simulink model "aeroblk_HL20_UE"  (R2023a)
settings: Solver=ode45  StartTime=0.0  StopTime=70  RelTol=1e-3  EnableMultiTasking=on
PreLoadFcn:
  | aeroblk_init_HL20
values from neighbouring files (symbols this model uses):
  Act2Aero = 0.5*[1 -1 0 0 0 0 0;1 1 0 0 0 0 0 ;0 0 0 0 0 0 2;0 0 1 1 0 0 0; 0 0 0 0 1 1 0;0 0 1 -1 1 -1 0;]    [aeroblk_init_HL20.m]
  Aero2Act = pinv(Act2Aero)    [aeroblk_init_HL20.m]
  Aimpoint = 0    [aeroblk_init_HL20.m]
undefined symbols (not defined in the file or in its folder): alpha0, ft, hglide, m, qbar0, s, U_trim_matrix, Xglide
libraries: aerolibconvert2 x11, aeroblk_lib_HL20 x5, simulink x2, aerolibactuator x1, aerolibsim3d x1, sim3dlib x1
Description:
  | HL-20 with Simulink 3D Animation and Flight Instrumentation Blocks
  | 
  | This model shows NASA's HL-20 lifting body and controller modeled in Simulink(R),
  |  Aerospace Blockset(TM), and Simulink(R) 3D Animation(TM) software. This model simulates
  | approach and landing flight phases using an auto-landing controller. The Visualization subsystem uses
  | aircraft-specific gauges from the Aerospace Blockset(TM) Flight Instrumentation library.
  | 
  | The HL-20 also known as personnel launch system (PLS) is a lifting body re-entry
  | vehicle that was designed to complement the Space Shuttle orbiter. Designed to
  | carry up to ten people and very little cargo[1], the HL-20 lifting body was to be
  | placed in orbit either launched vertically via booster rockets or transported in the
  | payload bay of the Space Shuttle orbiter. HL-20 lifting body was designed to have a
  | powered deorbiting accomplished with an onboard propulsion system while its reentry
  | was to be nose-first, horizontal and unpowered.
  | 
  | The HL-20 lifting body was developed as a low cost solution for getting to and from
  | low Earth orbit. The proposed benefits of the HL-20 were reduced operating costs
  | due to rapid turnaround between landing and launch, improved flight safety, and
  | ability to land conventionally on runways. Potential scenarios for the HL-20 were
  | orbital rescue of stranded astronauts, International Space Station crew exchange
  | if the Space Shuttle orbiter was not available, observation missions, and satellite
  | servicing missions.
  | 
  | Additional information about HL-20
  | 
  | [1] Jackson E. B., Cruz C. L., "Preliminary Subsonic Aerodynamic Model for Simulation Studies of the HL-20 Lifting Body," NASA TM4302 (August 1992)
settings Model: ModifiedByFormat=rhyde  ModifiedComment=rhyde -- Wed Mar 13 13:42:21 2002 -- Version 1.0  ModifiedHistory=A.N.Other -- Wed Mar 13 13:42:21 2002 -- Version 1.0  Creator=The MathWorks, Inc.  LastModifiedBy=rhyde
settings SolverCC: AlgebraicLoopSolver=TrustRegion  MaxZcPerStep=1
settings DataIOCC: LimitDataPoints=on  SaveFormat=Array  ReturnWorkspaceOutputs=off  SignalLoggingName=sigsOut
settings OptimizationCC: DefaultParameterBehavior=Inlined  InlineInvariantSignals=on  ReuseModelBlockBuffer=off  ExpressionDepthLimit=2147483647  InitFltsAndDblsToZero=on  EfficientFloat2IntCast=on  LifeSpan=inf
settings DebuggingCC: SaveWithParameterizedLinksMsg=none  CheckExecutionContextPreStartOutputMsg=on  MultiTaskCondExecSysMsg=none  SigSpecEnsureSampleTimeMsg=none  FcnCallInpInsideContextMsg=warning  UnconnectedInputMsg=warning  UnconnectedOutputMsg=warning  UnconnectedLineMsg=warning  UniqueDataStoreMsg=error  AllowSymbolicDim=off  StateNameClashWarn=warning  StrictBusMsg=ErrorOnBusTreatedAsVector  SFUnexpectedBacktrackingDiag=warning  SFNoUnconditionalDefaultTransitionDiag=warning  SFExecutionAtInitializationDiag=none  ArithmeticOperatorsInVariantConditions=warning
settings HardwareCC: ProdBitPerPointer=32  ProdBitPerSizeT=32  ProdBitPerPtrDiffT=32  ProdLargestAtomicFloat=None  ProdIntDivRoundTo=Undefined  ProdEndianess=Unspecified  ProdWordSize=32  ProdHWDeviceType=32-bit Generic  TargetUnknown=on
settings ModelReferenceCC: EnableRefExpFcnMdlSchedulingChecks=on  PropagateSignalLabelsOutOfModel=off
settings SFSimCC: SimUseLocalCustomCode=off  CustomCodeUndefinedFunction=UseInterfaceOnly
settings RTWCC: RTWUseLocalCustomCode=off  DLArmComputeVersion=19.05
settings CodeAppCC: StateflowObjectComments=on
settings GRTTargetCC: TargetFcnLib=ansi_tfl_tmw.mat  TargetLangStandard=C89/C90 (ANSI)  CombineOutputUpdateFcns=off  GRTInterface=on
settings ConfigComp: CovMetricSettings=dw  CovSaveCumulativeToWorkspaceVar=on  CovSaveSingleToWorkspaceVar=on  CovExternalEMLEnable=off

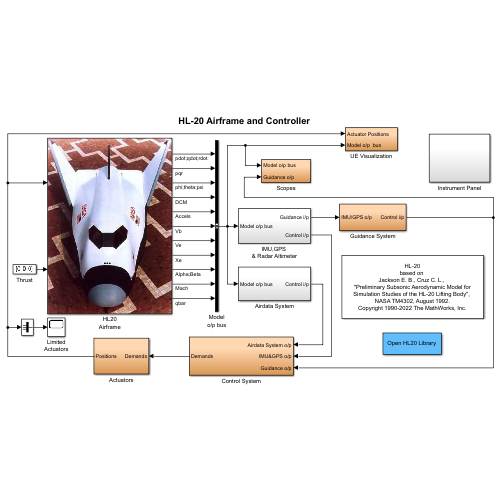
[thumbnail: Simulink's stored preview of the top-level diagram]
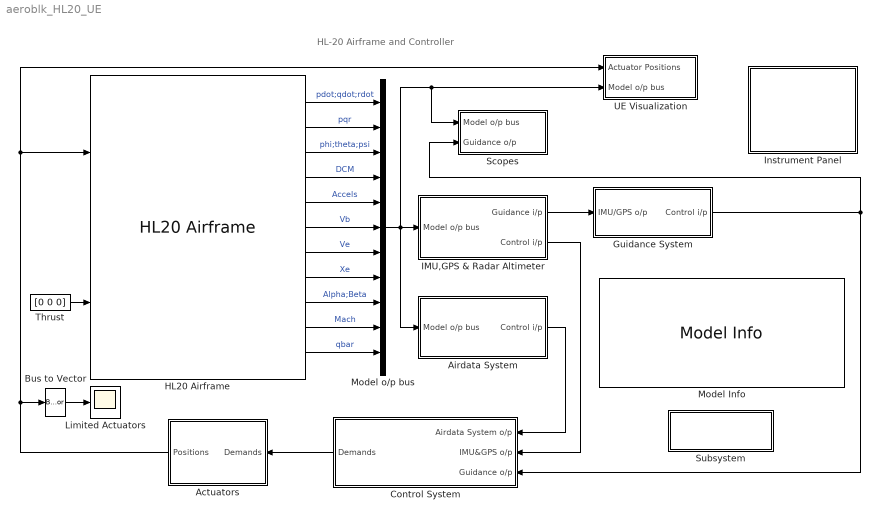
== system aeroblk_HL20_UE ==
  note: HL-20 Airframe and Controller
  Actuators : Subsystem
  Airdata System : Subsystem
  Bus to Vector : BusToVector
  Control System : Subsystem
  Guidance System : Subsystem
  HL20 Airframe : aeroblk_lib_HL20/HL20 Airframe  SystemSampleTime=-1  VariantActivationTime=update diagram  Latency=0  AutoFrameSizeCalculation=off
  IMU,GPS & Radar Altimeter : Subsystem
  Instrument Panel : Subsystem
  Limited Actuators : Scope
  Model o/p bus : BusCreator  Inputs=11
  Model Info : simulink/Model-Wide Utilities/Model Info  Frame=on  DisplayStringWithTags=|  HorizontalTextAlignment=Center  LeftAlignmentValue=0.5
      | HL-20
      | based on 
      | Jackson E. B., Cruz C. L., 
      | "Preliminary Subsonic Aerodynamic Model for
      | Simulation Studies of the HL-20 Lifting Body", 
      | NASA TM4302, August 1992.
      | Copyright 1990-2022 The MathWorks, Inc.
  Scopes : Subsystem
  Subsystem : Subsystem
      settings: OpenFcn=aeroblk_lib_HL20
      mask Display: disp('Open HL20 Library')
  Thrust : Constant  Value=[0 0 0]
  UE Visualization : Subsystem
  wires:
  Thrust/1 -> HL20 Airframe/2
  Actuators/1(Positions) -> UE Visualization/1(Actuator Positions), HL20 Airframe/1, Bus to Vector/1
  Guidance System/1(Control i/p) -> Scopes/2(Guidance o/p), Control System/3(Guidance o/p)
  Control System/1(Demands) -> Actuators/1(Demands)
  HL20 Airframe/1 -> Model o/p bus/1  "pdot;qdot;rdot"
  HL20 Airframe/2 -> Model o/p bus/2  "pqr"
  HL20 Airframe/3 -> Model o/p bus/3  "phi;theta;psi"
  HL20 Airframe/4 -> Model o/p bus/4  "DCM"
  HL20 Airframe/5 -> Model o/p bus/5  "Accels"
  HL20 Airframe/6 -> Model o/p bus/6  "Vb"
  HL20 Airframe/7 -> Model o/p bus/7  "Ve"
  HL20 Airframe/8 -> Model o/p bus/8  "Xe"
  HL20 Airframe/9 -> Model o/p bus/9  "Alpha;Beta"
  HL20 Airframe/10 -> Model o/p bus/10  "Mach"
  HL20 Airframe/11 -> Model o/p bus/11  "qbar"
  Model o/p bus/1 -> UE Visualization/2(Model o/p bus), Scopes/1(Model o/p bus), IMU,GPS & Radar Altimeter/1(Model o/p bus), Airdata System/1(Model o/p bus)
  IMU,GPS & Radar Altimeter/2(Control i/p) -> Control System/2(IMU&GPS o/p)
  Airdata System/1(Control i/p) -> Control System/1(Airdata System o/p)
  IMU,GPS & Radar Altimeter/1(Guidance i/p) -> Guidance System/1(IMU/GPS o/p)
  Bus to Vector/1 -> Limited Actuators/1

== system aeroblk_HL20_UE/Actuators ==
  Demands : Inport
  Act2Aero : Gain  Gain=Act2Aero  Multiplication=Matrix(K*u)  SaturateOnIntegerOverflow=on  OutDataTypeStr=Inherit: Same as input  ParamDataTypeStr=Inherit: Same as input
  Aero2Act : Gain  Gain=Aero2Act  Multiplication=Matrix(K*u)  SaturateOnIntegerOverflow=on  OutDataTypeStr=Inherit: Same as input  ParamDataTypeStr=Inherit: Same as input
  Bus Creator1 : BusCreator  Inputs=6
  Demux : Demux  Outputs=6
      settings: DisplayOption=none
  Nonlinear Second-Order Actuator : aerolibactuator/Nonlinear Second-Order Actuator  wn_fin=wn_act  z_fin=z_act  fin_max=max_lim  fin_min=min_lim  fin_maxrate=inf  fin_act_0=0  fin_act_vel=0
  Positions : Outport  VectorParamsAs1DForOutWhenUnconnected=off
  wires:
  Demands/1 -> Aero2Act/1
  Act2Aero/1 -> Demux/1
  Aero2Act/1 -> Nonlinear Second-Order Actuator/1
  Nonlinear Second-Order Actuator/1 -> Act2Aero/1
  Bus Creator1/1 -> Positions/1
  Demux/6 -> Bus Creator1/6  "Flap(diff)"
  Demux/5 -> Bus Creator1/5  "Flap(neg)"
  Demux/4 -> Bus Creator1/4  "Flap(pos)"
  Demux/3 -> Bus Creator1/3  "Rudder"
  Demux/2 -> Bus Creator1/2  "Elevator"
  Demux/1 -> Bus Creator1/1  "Aileron"

== system aeroblk_HL20_UE/Airdata System ==
  Model o/p bus : Inport
  Bus Creator1 : BusCreator  Inputs=2
  Bus Selector : BusSelector  OutputSignals=Alpha;Beta,qbar
  Control i/p : Outport  VectorParamsAs1DForOutWhenUnconnected=off
  wires:
  Model o/p bus/1 -> Bus Selector/1
  Bus Selector/1 -> Bus Creator1/1  "<Alpha;Beta>"
  Bus Selector/2 -> Bus Creator1/2  "<qbar>"
  Bus Creator1/1 -> Control i/p/1

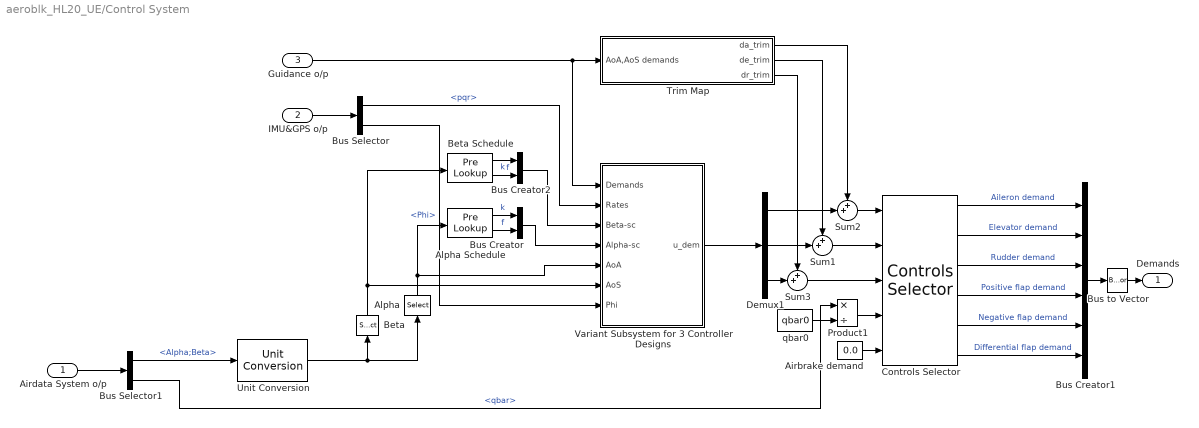
== system aeroblk_HL20_UE/Control System ==
  Airdata System o/p : Inport
  IMU&GPS o/p : Inport  Port=2
  Guidance o/p : Inport  Port=3
  Airbrake demand : Constant  Value=0.0
  Alpha : Selector  IndexMode=Zero-based  InputPortWidth=2  IndexOptions=Index vector (dialog)  Indices=0  OutputSizes=1
  Alpha Schedule : PreLookup  BreakpointsData=a_vec  BeginIndexSearchUsingPreviousIndexResult=on  ExtrapMethod=Linear
  Beta : Selector  IndexMode=Zero-based  InputPortWidth=2  IndexOptions=Index vector (dialog)  Indices=1  OutputSizes=1
  Beta Schedule : PreLookup  BreakpointsData=b_vec  BeginIndexSearchUsingPreviousIndexResult=on  ExtrapMethod=Linear
  Bus Creator : BusCreator  Inputs=2
  Bus Creator1 : BusCreator  Inputs=6
  Bus Creator2 : BusCreator  Inputs=2
  Bus Selector : BusSelector  OutputSignals=pqr,Phi
  Bus Selector1 : BusSelector  OutputSignals=Alpha;Beta,qbar
  Bus to Vector : BusToVector
  Controls Selector : aeroblk_lib_HL20/Controls Selector  SystemSampleTime=-1  VariantActivationTime=update diagram  Latency=0  AutoFrameSizeCalculation=off
  Demux1 : Demux  Outputs=3
      settings: DisplayOption=none
  Product1 : Product  Inputs=*/  InputSameDT=on  SaturateOnIntegerOverflow=on  OutDataTypeStr=Inherit: Same as first input
  Sum1 : Sum  Inputs=++|  InputSameDT=on  SaturateOnIntegerOverflow=on  OutDataTypeStr=Inherit: Same as first input
  Sum2 : Sum  Inputs=++|  InputSameDT=on  SaturateOnIntegerOverflow=on  OutDataTypeStr=Inherit: Same as first input
  Sum3 : Sum  Inputs=++|  InputSameDT=on  SaturateOnIntegerOverflow=on  OutDataTypeStr=Inherit: Same as first input
  Trim Map : Subsystem
  Unit Conversion : UnitConversion
  Variant Subsystem for 3 Controller Designs : Subsystem  Variant=on  VariantControlMode=label  LabelModeActiveChoice=ClassicalController
  qbar0 : Constant  Value=qbar0
  Demands : Outport  VectorParamsAs1DForOutWhenUnconnected=off
  wires:
  Bus to Vector/1 -> Demands/1
  Airbrake demand/1 -> Controls Selector/5
  Bus Selector1/2 -> Product1/1  "<qbar>"
  Bus Selector1/1 -> Unit Conversion/1  "<Alpha;Beta>"
  Airdata System o/p/1 -> Bus Selector1/1
  Bus Selector/2 -> Variant Subsystem for 3 Controller Designs/7(Phi)  "<Phi>"
  IMU&GPS o/p/1 -> Bus Selector/1
  Variant Subsystem for 3 Controller Designs/1(u_dem) -> Demux1/1
  Demux1/1 -> Sum2/2
  Demux1/3 -> Sum3/2
  Demux1/2 -> Sum1/2
  Trim Map/3(dr_trim) -> Sum3/1
  Trim Map/2(de_trim) -> Sum1/1
  Sum3/1 -> Controls Selector/3
  Sum1/1 -> Controls Selector/2
  Trim Map/1(da_trim) -> Sum2/1
  Sum2/1 -> Controls Selector/1
  qbar0/1 -> Product1/2
  Product1/1 -> Controls Selector/4
  Beta/1 -> Variant Subsystem for 3 Controller Designs/6(AoS), Beta Schedule/1
  Controls Selector/6 -> Bus Creator1/6  "Differential flap demand"
  Controls Selector/5 -> Bus Creator1/5  "Negative flap demand"
  Controls Selector/4 -> Bus Creator1/4  "Positive flap demand"
  Controls Selector/3 -> Bus Creator1/3  "Rudder demand"
  Controls Selector/2 -> Bus Creator1/2  "Elevator demand"
  Controls Selector/1 -> Bus Creator1/1  "Aileron demand"
  Unit Conversion/1 -> Alpha/1, Beta/1
  Alpha/1 -> Variant Subsystem for 3 Controller Designs/5(AoA), Alpha Schedule/1
  Guidance o/p/1 -> Variant Subsystem for 3 Controller Designs/1(Demands), Trim Map/1(AoA,AoS demands)
  Bus Selector/1 -> Variant Subsystem for 3 Controller Designs/2(Rates)  "<pqr>"
  Bus Creator2/1 -> Variant Subsystem for 3 Controller Designs/3(Beta-sc)
  Bus Creator/1 -> Variant Subsystem for 3 Controller Designs/4(Alpha-sc)
  Bus Creator1/1 -> Bus to Vector/1
  Alpha Schedule/1 -> Bus Creator/1  "k"
  Alpha Schedule/2 -> Bus Creator/2  "f"
  Beta Schedule/1 -> Bus Creator2/1  "k"
  Beta Schedule/2 -> Bus Creator2/2  "f"

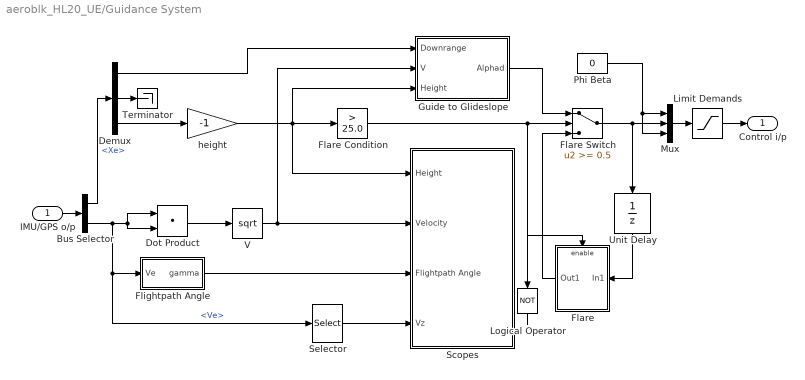
== system aeroblk_HL20_UE/Guidance System ==
  IMU/GPS o/p : Inport
  Bus Selector : BusSelector  OutputSignals=Xe,Ve
  Demux : Demux  Outputs=3
      settings: DisplayOption=none
  Dot Product : DotProduct  SaturateOnIntegerOverflow=on  InputSameDT=off  OutDataTypeStr=Inherit: Inherit via internal rule
  Flare : Subsystem  TreatAsAtomicUnit=on
  Flare Condition : simulink/Logic and Bit Operations/Compare To Constant  relop=>  const=25.0  OutDataTypeStr=boolean  ZeroCross=off
  Flare Switch : Switch  Threshold=0.5
  Flightpath Angle : Subsystem
  Guide to Glideslope : Subsystem
  Limit Demands : Saturate  UpperLimit=[20 25 5]  LowerLimit=[-20 -10 -5]
  Logical Operator : Logic  Operator=NOT
  Mux : Mux  Inputs=3
  Phi Beta : Constant  Value=0
  Scopes : Subsystem
  Selector : Selector  IndexMode=Zero-based  InputPortWidth=3  IndexOptions=Index vector (dialog)  Indices=2  OutputSizes=1
  Terminator : Terminator
  Unit Delay : UnitDelay  SampleTime=0.1  HasFrameUpgradeWarning=on
  V : Sqrt
  height : Gain  Gain=-1  SaturateOnIntegerOverflow=on  OutDataTypeStr=Inherit: Same as input  ParamDataTypeStr=Inherit: Same as input
  Control i/p : Outport  VectorParamsAs1DForOutWhenUnconnected=off
  wires:
  IMU/GPS o/p/1 -> Bus Selector/1
  Bus Selector/2 -> Selector/1, Flightpath Angle/1(Ve), Dot Product/1, Dot Product/2  "<Ve>"
  Flightpath Angle/1(gamma) -> Scopes/3(Flightpath Angle)
  Bus Selector/1 -> Demux/1  "<Xe>"
  Demux/1 -> Guide to Glideslope/1(Downrange)
  Demux/3 -> height/1
  height/1 -> Flare Condition/1, Guide to Glideslope/3(Height), Scopes/1(Height)
  Mux/1 -> Limit Demands/1
  V/1 -> Guide to Glideslope/2(V), Scopes/2(Velocity)
  Selector/1 -> Scopes/4(Vz)
  Phi Beta/1 -> Mux/3, Mux/1
  Flare Condition/1 -> Flare Switch/2, Logical Operator/1
  Flare Switch/1 -> Mux/2, Unit Delay/1
  Flare/1(Out1) -> Flare Switch/3
  Limit Demands/1 -> Control i/p/1
  Guide to Glideslope/1(Alphad) -> Flare Switch/1
  Demux/2 -> Terminator/1
  Logical Operator/1 -> Flare/Enable
  Unit Delay/1 -> Flare/1(In1)
  Dot Product/1 -> V/1

== system aeroblk_HL20_UE/IMU,GPS & Radar Altimeter ==
  Model o/p bus : Inport
  Bus Creator : BusCreator  Inputs=7
  Bus Creator1 : BusCreator  Inputs=2
  Bus Selector : BusSelector  OutputSignals=pqr,phi;theta;psi,DCM,Accels,Vb,Ve,Xe
  Select Phi : Selector  IndexMode=Zero-based  InputPortWidth=3  IndexOptions=Index vector (dialog)  Indices=0  OutputSizes=1
  Guidance i/p : Outport  VectorParamsAs1DForOutWhenUnconnected=off
  Control i/p : Outport  Port=2  VectorParamsAs1DForOutWhenUnconnected=off
  wires:
  Model o/p bus/1 -> Bus Selector/1
  Bus Selector/1 -> Bus Creator/1, Bus Creator1/1  "<pqr>"
  Bus Selector/2 -> Bus Creator/2, Select Phi/1  "<phi;theta;psi>"
  Bus Selector/3 -> Bus Creator/3  "<DCM>"
  Bus Selector/4 -> Bus Creator/4  "<Accels>"
  Bus Selector/5 -> Bus Creator/5  "<Vb>"
  Bus Selector/6 -> Bus Creator/6  "<Ve>"
  Bus Selector/7 -> Bus Creator/7  "<Xe>"
  Bus Creator/1 -> Guidance i/p/1
  Select Phi/1 -> Bus Creator1/2  "Phi"
  Bus Creator1/1 -> Control i/p/1

== system aeroblk_HL20_UE/Instrument Panel ==
  Airspeed Indicator : AirspeedIndicatorBlock  LabelPosition=Hide  ScaleMin=0  ScaleMax=450
  Altimeter : AltimeterBlock  LabelPosition=Hide
  Artificial Horizon : ArtificialHorizonBlock  LabelPosition=Hide
  Climb Rate Indicator : ClimbIndicatorBlock  LabelPosition=Hide  ScaleMax=16000
  Heading Indicator : HeadingIndicatorBlock  LabelPosition=Hide
  Turn Coordinator : TurnCoordinatorBlock  LabelPosition=Hide

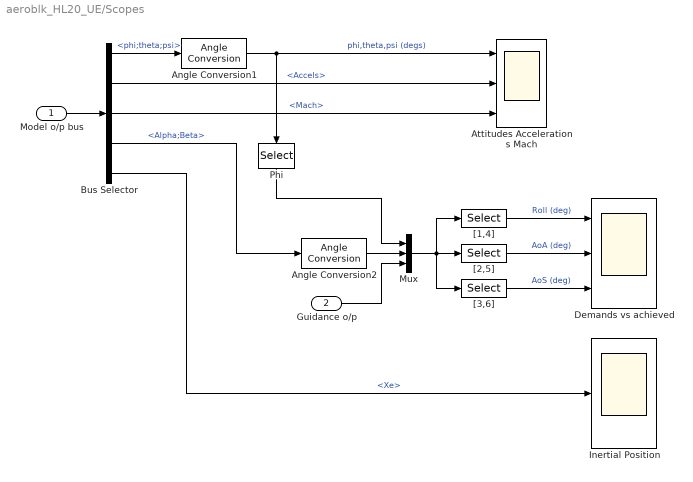
== system aeroblk_HL20_UE/Scopes ==
  Model o/p bus : Inport
  Guidance o/p : Inport  Port=2
  Angle Conversion1 : aerolibconvert2/Angle Conversion  IU=rad  OU=deg
  Angle Conversion2 : aerolibconvert2/Angle Conversion  IU=rad  OU=deg
  Attitudes Accelerations Mach : Scope  NumInputPorts=3
  Bus Selector : BusSelector  OutputSignals=phi;theta;psi,Accels,Mach,Alpha;Beta,Xe
  Demands vs achieved : Scope  NumInputPorts=3
  Inertial Position : Scope
  Mux : Mux  Inputs=[1,2,3]
  Phi : Selector  IndexMode=Zero-based  InputPortWidth=3  IndexOptions=Index vector (dialog)  Indices=0  OutputSizes=1
  "[1,4]" : Selector  IndexMode=Zero-based  InputPortWidth=6  IndexOptions=Index vector (dialog)  Indices=[0 3]  OutputSizes=1
  "[2,5]" : Selector  IndexMode=Zero-based  InputPortWidth=6  IndexOptions=Index vector (dialog)  Indices=[1 4]  OutputSizes=1
  "[3,6]" : Selector  IndexMode=Zero-based  InputPortWidth=6  IndexOptions=Index vector (dialog)  Indices=[2 5]  OutputSizes=1
  wires:
  Model o/p bus/1 -> Bus Selector/1
  Bus Selector/1 -> Angle Conversion1/1  "<phi;theta;psi>"
  Bus Selector/2 -> Attitudes Accelerations Mach/2  "<Accels>"
  Bus Selector/3 -> Attitudes Accelerations Mach/3  "<Mach>"
  Phi/1 -> Mux/1
  Bus Selector/4 -> Angle Conversion2/1  "<Alpha;Beta>"
  Angle Conversion2/1 -> Mux/2
  Mux/1 -> "[2,5]"/1, "[3,6]"/1, "[1,4]"/1
  Guidance o/p/1 -> Mux/3
  "[1,4]"/1 -> Demands vs achieved/1  "Roll (deg)"
  "[2,5]"/1 -> Demands vs achieved/2  "AoA (deg)"
  "[3,6]"/1 -> Demands vs achieved/3  "AoS (deg)"
  Bus Selector/5 -> Inertial Position/1  "<Xe>"
  Angle Conversion1/1 -> Phi/1, Attitudes Accelerations Mach/1  "phi,theta,psi (degs)"

== system aeroblk_HL20_UE/Subsystem ==

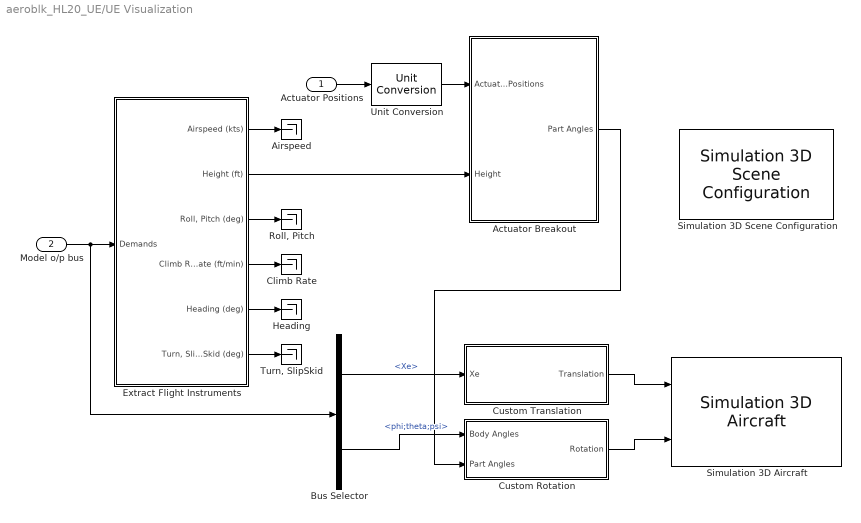
== system aeroblk_HL20_UE/UE Visualization ==
  Actuator Positions : Inport  Unit=deg
  Model o/p bus : Inport  Port=2
  Actuator Breakout : Subsystem
  Airspeed : Terminator
  Bus Selector : BusSelector  OutputSignals=Xe,phi;theta;psi
  Climb Rate : Terminator
  Custom Rotation : Subsystem
  Custom Translation : Subsystem
  Extract Flight Instruments : Subsystem
  Heading : Terminator
  "Roll, Pitch" : Terminator
  Simulation 3D Aircraft : aerolibsim3d/Simulation 3D Aircraft  Priority=-1  Mesh=Custom  MeshPath=/MathWorksAerospaceContent/Vehicles/Aircraft/Custom/Mesh/SK_HL20.SK_HL20  MeshPathAT=/MathWorksAerospaceContent/Vehicles/Aircraft/AirTransport/Mesh/SK_AirTransport.SK_AirTransport  MeshPathGA=/MathWorksAerospaceContent/Vehicles/Aircraft/GeneralAviation/Mesh/SK_GeneralAviation.SK_GeneralAviation  AircraftColor=White  ActorName=SimulinkHL20  Translation=[-7000, 0, -3048; zeros( 56, 3 )]  Rotation=zeros( 57, 3 )  IsGHSensorEnabled=off  AreGHRaysVisible=off  IsOutputReshapeEnabled=off  GHRayLength=5000  GHBodyOffset=0.90  GHFrontTireRadius=0.21  GHLeftTireRadius=0.21  GHRightTireRadius=0.21  WoWSensorTolerance=0.05  LightsConfig=Automatic lights  LandingLightIntensity=300000  LandingLightConeAngle=15  CustomLeftLandingLightLocation=[0 0 0]  CustomLeftLandingLightOrientation=[0 0 0]  CustomRightLandingLightLocation=[0 0 0]  CustomRightLandingLightOrientation=[0 0 0]  TaxiLightIntensity=150000  TaxiLightConeAngle=36  CustomTaxiLightLocation=[0 0 0]  CustomTaxiLightOrientation=[0 0 0]  NavLightIntensity=500  PositionLightIntensity=500  StrobeLightIntensity=5000  WingtipStrobePeriod=1.5  WingtipStrobePulseWidth=6  TailStrobePeriod=1.5  TailStrobePulseWidth=6  BeaconLightIntensity=4000  BeaconPeriod=1.5  BeaconPulseWidth=10  SampleTime=-1  ActorType=SimulinkVehicle  ID=C  aMode=0  ActorTag=SimulinkHL20
  Simulation 3D Scene Configuration : sim3dlib/Simulation 3D Scene Configuration  Priority=0  ProjectFormat=Default Scenes  SceneDesc=Airport  ProjectName=B:\matlab\toolbox\shared\sim3d_projects\automotive_project\UE4\WindowsNoEditor\VehicleSimulation.exe  ScenePath=/Game/Maps/HwStrght  EnableOpenDRIVE=off  vehTagList={'Scene Origin';'SimulinkHL20'}  vehTag=SimulinkHL20  OpVisEn=off  Ts=1/60  EnableWindow=on  EnableRemoteAccess=off  EnableWeather=off  SunAltitude=40.0  SunAzimuth=90  clouds=10  wind=1  fog=0  rain=0  EnableGeospatial=off  OriginHeight=200  OriginLatitude=40.744652  OriginLongitude=-73.988864  MapStyle=Aerial  AdditionalAssetIDs=[]  UseAdvancedSunSky=off  SolarTime=11  TimeZone=-5  Day=21  Month=9  Year=2022  UseDaylightSavingTime=on  DSTStartDay=10  DSTStartMonth=3  DSTEndDay=3  DSTEndMonth=11  DSTSwitchHour=2  sensorTag=MainCamera1  sensorId=1  sensorName=MainCamera1  mountLoc=Origin  offsetFlag=off  tmountOffset=[0, 0, 0]  rmountOffset=[0, 0, 0]  HorizontalResolution=1280  VerticalResolution=720  HorizontalFOV=60  mountPoint=[0 0 0]  mountOrientation=[0 0 0]  aMode=0  ID=1  GeoTrigger=Inactive
      settings: LibrarySourceBlock=aerolibsim3d/Simulation 3D Scene Configuration
  "Turn, SlipSkid" : Terminator
  Unit Conversion : UnitConversion
  wires:
  Model o/p bus/1 -> Bus Selector/1, Extract Flight Instruments/1(Demands)
  Extract Flight Instruments/1(Airspeed (kts)) -> Airspeed/1
  Extract Flight Instruments/4(Climb Rate (ft/min)) -> Climb Rate/1
  Extract Flight Instruments/3("Roll, Pitch (deg)") -> "Roll, Pitch"/1
  Extract Flight Instruments/5(Heading (deg)) -> Heading/1
  Extract Flight Instruments/6("Turn, SlipSkid (deg)") -> "Turn, SlipSkid"/1
  Custom Rotation/1(Rotation) -> Simulation 3D Aircraft/2
  Custom Translation/1(Translation) -> Simulation 3D Aircraft/1
  Bus Selector/1 -> Custom Translation/1(Xe)  "<Xe>"
  Bus Selector/2 -> Custom Rotation/1(Body Angles)  "<phi;theta;psi>"
  Extract Flight Instruments/2(Height (ft)) -> Actuator Breakout/2(Height)
  Actuator Breakout/1(Part Angles) -> Custom Rotation/2(Part Angles)
  Actuator Positions/1 -> Unit Conversion/1
  Unit Conversion/1 -> Actuator Breakout/1(Actuator Positions)

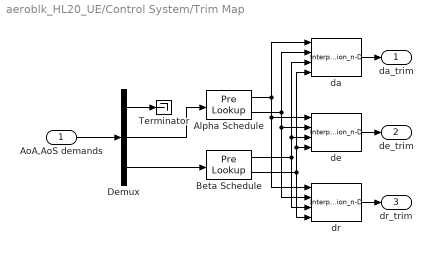
== system aeroblk_HL20_UE/Control System/Trim Map ==
  AoA,AoS demands : Inport
  Alpha Schedule : PreLookup  BreakpointsData=a_vec  BeginIndexSearchUsingPreviousIndexResult=on  ExtrapMethod=Linear
  Beta Schedule : PreLookup  BreakpointsData=b_vec  BeginIndexSearchUsingPreviousIndexResult=on  ExtrapMethod=Linear
  Demux : Demux  Outputs=3
      settings: DisplayOption=none
  Terminator : Terminator
  da : Interpolation_n-D  Table=squeeze(U_trim_matrix(1,:,:))  RemoveProtectionIndex=on  SaturateOnIntegerOverflow=on
  de : Interpolation_n-D  Table=squeeze(U_trim_matrix(2,:,:))  RemoveProtectionIndex=on  SaturateOnIntegerOverflow=on
  dr : Interpolation_n-D  Table=squeeze(U_trim_matrix(3,:,:))  RemoveProtectionIndex=on  SaturateOnIntegerOverflow=on
  da_trim : Outport  VectorParamsAs1DForOutWhenUnconnected=off
  de_trim : Outport  Port=2  VectorParamsAs1DForOutWhenUnconnected=off
  dr_trim : Outport  Port=3  VectorParamsAs1DForOutWhenUnconnected=off
  wires:
  dr/1 -> dr_trim/1
  de/1 -> de_trim/1
  da/1 -> da_trim/1
  Demux/1 -> Terminator/1
  Demux/3 -> Beta Schedule/1
  Demux/2 -> Alpha Schedule/1
  AoA,AoS demands/1 -> Demux/1
  Beta Schedule/1 -> da/3, de/3, dr/3
  Alpha Schedule/1 -> de/1, dr/1, da/1
  Alpha Schedule/2 -> da/2, de/2, dr/2
  Beta Schedule/2 -> da/4, de/4, dr/4

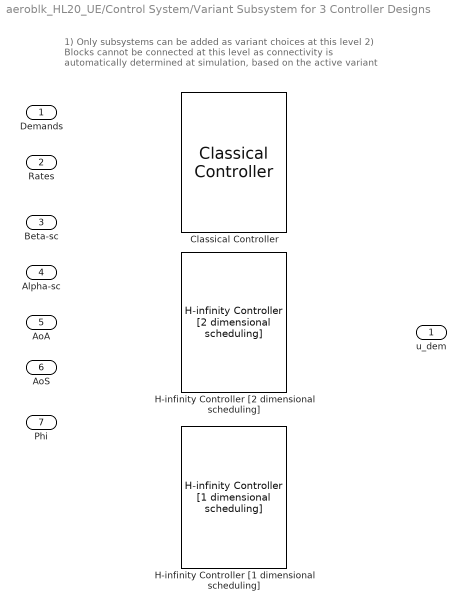
== system aeroblk_HL20_UE/Control System/Variant Subsystem for 3 Controller Designs ==
  note: 1) Only subsystems can be added as variant choices at this level
      | 2) Blocks cannot be connected at this level as connectivity is
      | automatically determined at simulation, based on the active variant
  Demands : Inport
  Rates : Inport  Port=2
  Beta-sc : Inport  Port=3
  Alpha-sc : Inport  Port=4
  AoA : Inport  Port=5
  AoS : Inport  Port=6
  Phi : Inport  Port=7
  Classical Controller : aeroblk_lib_HL20/Classical Controller  SystemSampleTime=-1  VariantControl=ClassicalController  VariantActivationTime=update diagram  Latency=0  AutoFrameSizeCalculation=off
  H-infinity Controller [1 dimensional scheduling] : aeroblk_lib_HL20/H-infinity Controller [1 dimensional scheduling]  SystemSampleTime=-1  VariantControl=HInf1DimensionalController  VariantActivationTime=update diagram  Latency=0  AutoFrameSizeCalculation=off
  H-infinity Controller [2 dimensional scheduling] : aeroblk_lib_HL20/H-infinity Controller [2 dimensional scheduling]  SystemSampleTime=-1  VariantControl=HInf2DimensionalController  VariantActivationTime=update diagram  Latency=0  AutoFrameSizeCalculation=off
  u_dem : Outport  VectorParamsAs1DForOutWhenUnconnected=off

== system aeroblk_HL20_UE/Guidance System/Flare ==
  In1 : Inport
  Enable : EnablePort  StatesWhenEnabling=reset
  Alphad1 : Integrator  InitialConditionSource=external
  Flare Demand1 : Constant  Value=17.5
  Gain1 : Gain  Gain=2  SaturateOnIntegerOverflow=on  OutDataTypeStr=Inherit: Same as input  ParamDataTypeStr=Inherit: Same as input
  Sum2 : Sum  Inputs=|+-  InputSameDT=on  SaturateOnIntegerOverflow=on  OutDataTypeStr=Inherit: Same as first input
  Out1 : Outport  InitialOutput=[0]  VectorParamsAs1DForOutWhenUnconnected=off
  wires:
  In1/1 -> Alphad1/2
  Flare Demand1/1 -> Sum2/1
  Sum2/1 -> Gain1/1
  Gain1/1 -> Alphad1/1
  Alphad1/1 -> Sum2/2, Out1/1

== system aeroblk_HL20_UE/Guidance System/Flightpath Angle ==
  Ve : Inport
  Sum2 : Sum  Inputs=+  InputSameDT=on  SaturateOnIntegerOverflow=on  OutDataTypeStr=Inherit: Same as first input
  V : Sqrt
  product : Product  InputSameDT=on  SaturateOnIntegerOverflow=on  OutDataTypeStr=Inherit: Same as first input
  product1 : Product  Inputs=/*  InputSameDT=on  SaturateOnIntegerOverflow=on  OutDataTypeStr=Inherit: Same as first input
  rad-->deg4 : Gain  Gain=-1  SaturateOnIntegerOverflow=on  OutDataTypeStr=Inherit: Same as input  ParamDataTypeStr=Inherit: Same as input
  tangent : Trigonometry  Operator=atan
  u,v : Selector  IndexMode=Zero-based  InputPortWidth=3  IndexOptions=Index vector (dialog)  Indices=[0 1]  OutputSizes=1
  w : Selector  IndexMode=Zero-based  InputPortWidth=3  IndexOptions=Index vector (dialog)  Indices=2  OutputSizes=1
  gamma : Outport  VectorParamsAs1DForOutWhenUnconnected=off
  wires:
  tangent/1 -> gamma/1
  Ve/1 -> w/1, u,v/1
  product/1 -> Sum2/1
  Sum2/1 -> V/1
  product1/1 -> tangent/1
  rad-->deg4/1 -> product1/2
  V/1 -> product1/1
  u,v/1 -> product/2, product/1
  w/1 -> rad-->deg4/1

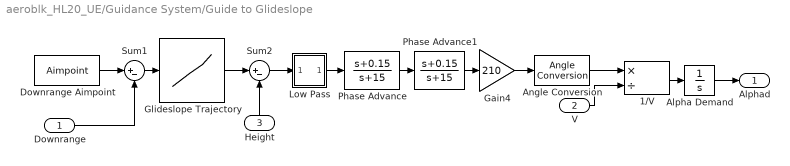
== system aeroblk_HL20_UE/Guidance System/Guide to Glideslope ==
  Downrange : Inport
  V : Inport  Port=2
  Height : Inport  Port=3
  1/V : Product  Inputs=*/  InputSameDT=on  SaturateOnIntegerOverflow=on  OutDataTypeStr=Inherit: Same as first input
  Alpha Demand : Integrator  InitialCondition=alpha0*180/pi
  Angle Conversion : aerolibconvert2/Angle Conversion  IU=rad  OU=deg
  Downrange Aimpoint : Constant  Value=Aimpoint
  Gain4 : Gain  Gain=210  SaturateOnIntegerOverflow=on  OutDataTypeStr=Inherit: Same as input  ParamDataTypeStr=Inherit: Same as input
  Glideslope Trajectory : Lookup_n-D  NumberOfTableDimensions=1  LookupTableObject=''  BreakpointsForDimension1=Xglide  Table=hglide  SaturateOnIntegerOverflow=on
  Low Pass : Subsystem
  Phase Advance : TransferFcn  Numerator=[1 0.15]  Denominator=[1 15]
  Phase Advance1 : TransferFcn  Numerator=[1 0.15]  Denominator=[1 15]
  Sum1 : Sum  Inputs=|+-  InputSameDT=on  SaturateOnIntegerOverflow=on  OutDataTypeStr=Inherit: Same as first input
  Sum2 : Sum  Inputs=|+-  InputSameDT=on  SaturateOnIntegerOverflow=on  OutDataTypeStr=Inherit: Same as first input
  Alphad : Outport  VectorParamsAs1DForOutWhenUnconnected=off
  wires:
  Downrange Aimpoint/1 -> Sum1/1
  Sum1/1 -> Glideslope Trajectory/1
  Glideslope Trajectory/1 -> Sum2/1
  Sum2/1 -> Low Pass/1(In1)
  Phase Advance1/1 -> Gain4/1
  Phase Advance/1 -> Phase Advance1/1
  Gain4/1 -> Angle Conversion/1
  1/V/1 -> Alpha Demand/1
  Low Pass/1(Out1) -> Phase Advance/1
  V/1 -> 1/V/2
  Height/1 -> Sum2/2
  Alpha Demand/1 -> Alphad/1
  Downrange/1 -> Sum1/2
  Angle Conversion/1 -> 1/V/1

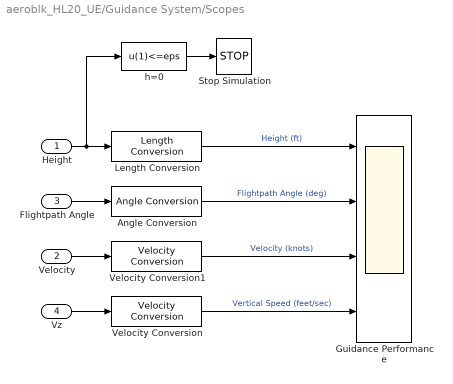
== system aeroblk_HL20_UE/Guidance System/Scopes ==
  Height : Inport
  Velocity : Inport  Port=2
  Flightpath Angle : Inport  Port=3
  Vz : Inport  Port=4
  Angle Conversion : aerolibconvert2/Angle Conversion  IU=rad  OU=deg
  Guidance Performance : Scope  NumInputPorts=4
  Length Conversion : aerolibconvert2/Length Conversion  IU=m  OU=ft
  Stop Simulation : Stop
  Velocity Conversion : aerolibconvert2/Velocity Conversion  IU=m/s  OU=ft/s
  Velocity Conversion1 : aerolibconvert2/Velocity Conversion  IU=m/s  OU=kts
  h=0 : Fcn  Expr=u(1)<=eps
  wires:
  Angle Conversion/1 -> Guidance Performance/2  "Flightpath Angle (deg)"
  Velocity Conversion/1 -> Guidance Performance/4  "Vertical Speed (feet/sec)"
  Velocity Conversion1/1 -> Guidance Performance/3  "Velocity (knots)"
  Length Conversion/1 -> Guidance Performance/1  "Height (ft)"
  Velocity/1 -> Velocity Conversion1/1
  Height/1 -> Length Conversion/1, h=0/1
  Flightpath Angle/1 -> Angle Conversion/1
  Vz/1 -> Velocity Conversion/1
  h=0/1 -> Stop Simulation/1

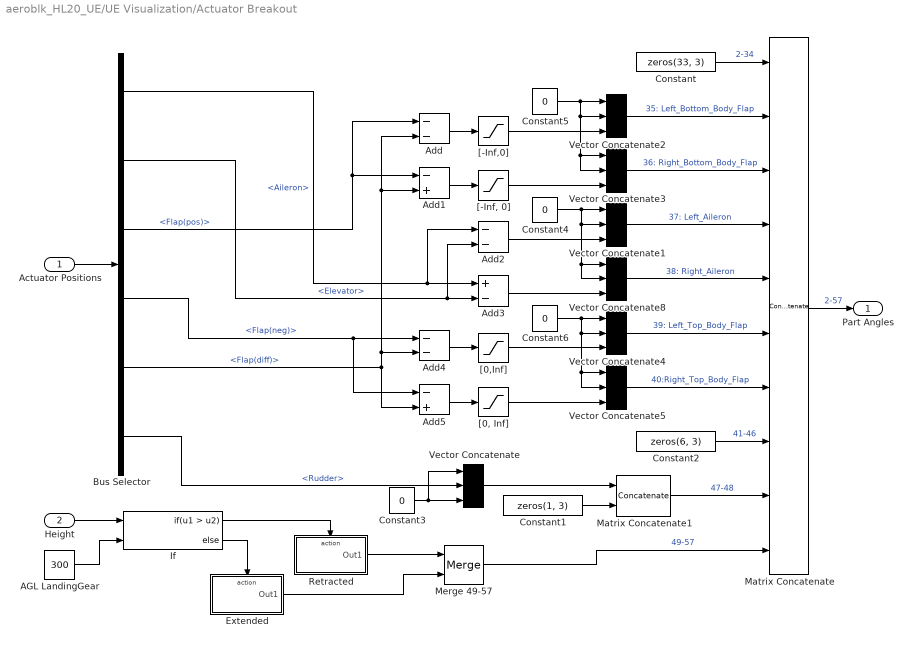
== system aeroblk_HL20_UE/UE Visualization/Actuator Breakout ==
  Actuator Positions : Inport  Unit=rad
  Height : Inport  Port=2
  AGL LandingGear : Constant  Value=300
  Add : Sum  Inputs=--
  Add1 : Sum  Inputs=-+
  Add2 : Sum  Inputs=--
  Add3 : Sum  Inputs=+-
  Add4 : Sum  Inputs=--
  Add5 : Sum  Inputs=-+
  Bus Selector : BusSelector  OutputSignals=Aileron,Elevator,Flap(pos),Flap(neg),Flap(diff),Rudder
  Constant : Constant  Value=zeros(33, 3)  VectorParams1D=off
  Constant1 : Constant  Value=zeros(1, 3)  VectorParams1D=off
  Constant2 : Constant  Value=zeros(6, 3)  VectorParams1D=off
  Constant{3..6} (4 alike) : Constant  Value=0
  Extended : Subsystem  TreatAsAtomicUnit=on
  If : If  NumInputs=2  IfExpression=u1 > u2
  Matrix Concatenate : Concatenate  NumInputs=10  Mode=Multidimensional array
  Matrix Concatenate1 : Concatenate  Mode=Multidimensional array
  Merge 49-57 : Merge  InitialOutput=[0 0 1.75;0 0 0;0 0 0;-2 0 0;0 0 0;0 0 0;2 0 0;0 0 0;0 0 0]
  Retracted : Subsystem  TreatAsAtomicUnit=on
  Vector Concatenate{,1..5,8} (7 alike) : Concatenate  NumInputs=3  Mode=Multidimensional array  ConcatenateDimension=2
  "[-Inf, 0]" : Saturate  UpperLimit=0  LowerLimit=-Inf
  "[-Inf,0]" : Saturate  UpperLimit=0  LowerLimit=-Inf
  "[0, Inf]" : Saturate  UpperLimit=Inf  LowerLimit=0
  "[0,Inf]" : Saturate  UpperLimit=Inf  LowerLimit=0
  Part Angles : Outport
  wires:
  AGL LandingGear/1 -> If/2
  Height/1 -> If/1
  If/1 -> Retracted/Action
  If/2 -> Extended/Action
  Actuator Positions/1 -> Bus Selector/1
  Matrix Concatenate/1 -> Part Angles/1  "2-57"
  Retracted/1(Out1) -> Merge 49-57/1
  Extended/1(Out1) -> Merge 49-57/2
  Constant/1 -> Matrix Concatenate/1  "2-34"
  Constant2/1 -> Matrix Concatenate/8  "41-46"
  Constant1/1 -> Matrix Concatenate1/2
  Merge 49-57/1 -> Matrix Concatenate/10  "49-57"
  Matrix Concatenate1/1 -> Matrix Concatenate/9  "47-48"
  Add4/1 -> "[0,Inf]"/1
  Add5/1 -> "[0, Inf]"/1
  Add/1 -> "[-Inf,0]"/1
  Add1/1 -> "[-Inf, 0]"/1
  Bus Selector/1 -> Add2/1, Add3/1  "<Aileron>"
  Bus Selector/2 -> Add2/2, Add3/2  "<Elevator>"
  Bus Selector/5 -> Add4/2, Add1/2, Add/2, Add5/2  "<Flap(diff)>"
  Vector Concatenate/1 -> Matrix Concatenate1/1
  Bus Selector/6 -> Vector Concatenate/2  "<Rudder>"
  Constant3/1 -> Vector Concatenate/3, Vector Concatenate/1
  Constant4/1 -> Vector Concatenate1/1, Vector Concatenate8/2, Vector Concatenate8/1, Vector Concatenate1/2
  Add2/1 -> Vector Concatenate1/3
  Add3/1 -> Vector Concatenate8/3
  Vector Concatenate1/1 -> Matrix Concatenate/4  "37: Left_Aileron"
  Vector Concatenate8/1 -> Matrix Concatenate/5  "38: Right_Aileron"
  "[-Inf,0]"/1 -> Vector Concatenate2/3
  Vector Concatenate2/1 -> Matrix Concatenate/2  "35: Left_Bottom_Body_Flap"
  "[-Inf, 0]"/1 -> Vector Concatenate3/3
  Vector Concatenate3/1 -> Matrix Concatenate/3  "36: Right_Bottom_Body_Flap"
  Constant5/1 -> Vector Concatenate3/2, Vector Concatenate3/1, Vector Concatenate2/2, Vector Concatenate2/1
  Vector Concatenate5/1 -> Matrix Concatenate/7  "40:Right_Top_Body_Flap"
  Vector Concatenate4/1 -> Matrix Concatenate/6  "39: Left_Top_Body_Flap"
  Constant6/1 -> Vector Concatenate4/1, Vector Concatenate4/2, Vector Concatenate5/1, Vector Concatenate5/2
  "[0,Inf]"/1 -> Vector Concatenate4/3
  "[0, Inf]"/1 -> Vector Concatenate5/3
  Bus Selector/3 -> Add1/1, Add/1  "<Flap(pos)>"
  Bus Selector/4 -> Add4/1, Add5/1  "<Flap(neg)>"

== system aeroblk_HL20_UE/UE Visualization/Custom Rotation ==
  note: phi; theta; psi]
  Body Angles : Inport  PortDimensions=[3, 1]
  Part Angles : Inport  Port=2
  Matrix Concatenate : Concatenate  Mode=Multidimensional array
  Reshape : Reshape  OutputDimensionality=Row vector (2-D)
  Rotation : Outport
  wires:
  Body Angles/1 -> Reshape/1
  Matrix Concatenate/1 -> Rotation/1
  Reshape/1 -> Matrix Concatenate/1
  Part Angles/1 -> Matrix Concatenate/2

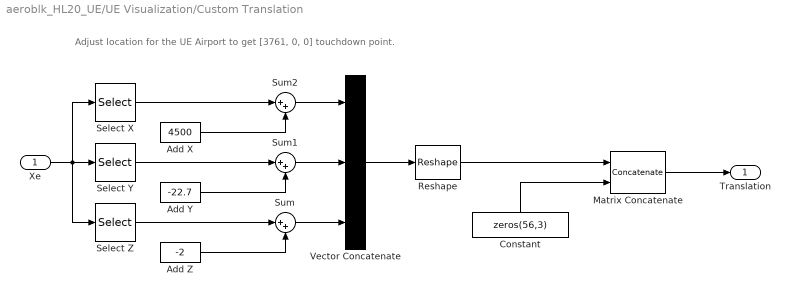
== system aeroblk_HL20_UE/UE Visualization/Custom Translation ==
  note: Adjust location for the UE Airport to get [3761, 0, 0] touchdown point.
  Xe : Inport
  Add X : Constant  Value=4500
  Add Y : Constant  Value=-22.7
  Add Z : Constant  Value=-2
  Constant : Constant  Value=zeros(56,3)
  Matrix Concatenate : Concatenate  Mode=Multidimensional array
  Reshape : Reshape  OutputDimensionality=Row vector (2-D)
  Select X : Selector  InputPortWidth=3  IndexOptions=Index vector (dialog)  Indices=1  OutputSizes=1
  Select Y : Selector  InputPortWidth=3  IndexOptions=Index vector (dialog)  Indices=2  OutputSizes=1
  Select Z : Selector  InputPortWidth=3  IndexOptions=Index vector (dialog)  Indices=3  OutputSizes=1
  Sum : Sum  Inputs=|++
  Sum1 : Sum  Inputs=|++
  Sum2 : Sum  Inputs=|++
  Vector Concatenate : Concatenate  NumInputs=3
  Translation : Outport
  wires:
  Matrix Concatenate/1 -> Translation/1
  Constant/1 -> Matrix Concatenate/2
  Reshape/1 -> Matrix Concatenate/1
  Xe/1 -> Select Y/1, Select Z/1, Select X/1
  Vector Concatenate/1 -> Reshape/1
  Sum/1 -> Vector Concatenate/3
  Select Z/1 -> Sum/1
  Add Z/1 -> Sum/2
  Sum1/1 -> Vector Concatenate/2
  Select Y/1 -> Sum1/1
  Add Y/1 -> Sum1/2
  Sum2/1 -> Vector Concatenate/1
  Select X/1 -> Sum2/1
  Add X/1 -> Sum2/2

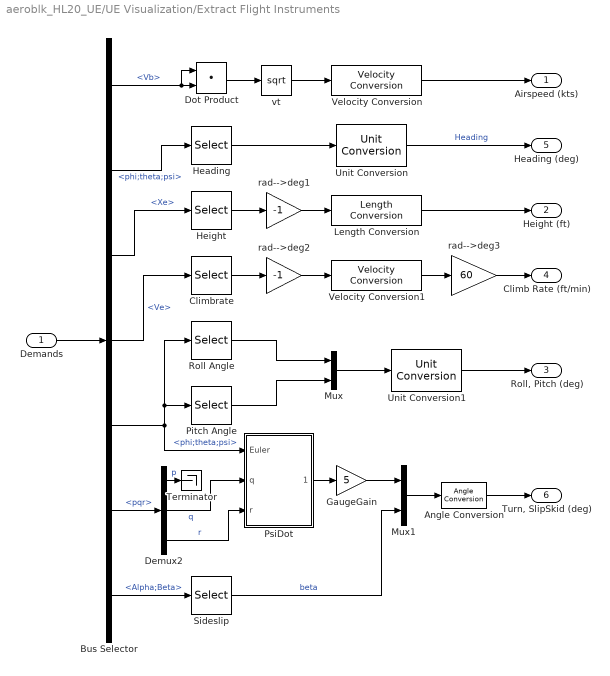
== system aeroblk_HL20_UE/UE Visualization/Extract Flight Instruments ==
  Demands : Inport
  Angle Conversion : aerolibconvert2/Angle Conversion  IU=rad  OU=deg
  Bus Selector : BusSelector  OutputSignals=Vb,phi;theta;psi,Xe,Ve,phi;theta;psi,pqr,Alpha;Beta
  Climbrate : Selector  IndexMode=Zero-based  InputPortWidth=3  IndexOptions=Index vector (dialog)  Indices=2  OutputSizes=1
  Demux2 : Demux  Outputs=3
  Dot Product : DotProduct  SaturateOnIntegerOverflow=on  InputSameDT=off  OutDataTypeStr=Inherit: Inherit via internal rule
  GaugeGain : Gain  Gain=5
  Heading : Selector  IndexMode=Zero-based  InputPortWidth=3  IndexOptions=Index vector (dialog)  Indices=2  OutputSizes=1
  Height : Selector  IndexMode=Zero-based  InputPortWidth=3  IndexOptions=Index vector (dialog)  Indices=2  OutputSizes=1
  Length Conversion : aerolibconvert2/Length Conversion  IU=m  OU=ft
  Mux : Mux  Inputs=2
  Mux1 : Mux  Inputs=2
  Pitch Angle : Selector  IndexMode=Zero-based  InputPortWidth=3  IndexOptions=Index vector (dialog)  Indices=1  OutputSizes=1
  PsiDot : Subsystem
  Roll Angle : Selector  IndexMode=Zero-based  InputPortWidth=3  IndexOptions=Index vector (dialog)  Indices=0  OutputSizes=1
  Sideslip : Selector  InputPortWidth=2  IndexOptions=Index vector (dialog)  Indices=2  OutputSizes=1
  Terminator : Terminator
  Unit Conversion : UnitConversion
  Unit Conversion1 : UnitConversion
  Velocity Conversion : aerolibconvert2/Velocity Conversion  IU=m/s  OU=kts
  Velocity Conversion1 : aerolibconvert2/Velocity Conversion  IU=m/s  OU=ft/s
  rad-->deg1 : Gain  Gain=-1  SaturateOnIntegerOverflow=on  OutDataTypeStr=Inherit: Same as input  ParamDataTypeStr=Inherit: Same as input
  rad-->deg2 : Gain  Gain=-1  SaturateOnIntegerOverflow=on  OutDataTypeStr=Inherit: Same as input  ParamDataTypeStr=Inherit: Same as input
  rad-->deg3 : Gain  Gain=60  SaturateOnIntegerOverflow=on  OutDataTypeStr=Inherit: Same as input  ParamDataTypeStr=Inherit: Same as input
  vt : Sqrt
  Airspeed (kts) : Outport  Unit=kn  VectorParamsAs1DForOutWhenUnconnected=off
  Height (ft) : Outport  Port=2  Unit=ft  VectorParamsAs1DForOutWhenUnconnected=off
  "Roll, Pitch (deg)" : Outport  Port=3  Unit=deg  VectorParamsAs1DForOutWhenUnconnected=off
  Climb Rate (ft/min) : Outport  Port=4  Unit=ft/min  VectorParamsAs1DForOutWhenUnconnected=off
  Heading (deg) : Outport  Port=5  Unit=deg  VectorParamsAs1DForOutWhenUnconnected=off
  "Turn, SlipSkid (deg)" : Outport  Port=6  Unit=deg  VectorParamsAs1DForOutWhenUnconnected=off
  wires:
  Unit Conversion1/1 -> "Roll, Pitch (deg)"/1
  Mux/1 -> Unit Conversion1/1
  Roll Angle/1 -> Mux/1
  rad-->deg3/1 -> Climb Rate (ft/min)/1
  Velocity Conversion1/1 -> rad-->deg3/1
  Bus Selector/4 -> Climbrate/1  "<Ve>"
  rad-->deg2/1 -> Velocity Conversion1/1
  Climbrate/1 -> rad-->deg2/1
  Length Conversion/1 -> Height (ft)/1
  rad-->deg1/1 -> Length Conversion/1
  Height/1 -> rad-->deg1/1
  Bus Selector/3 -> Height/1  "<Xe>"
  Unit Conversion/1 -> Heading (deg)/1  "Heading"
  Heading/1 -> Unit Conversion/1
  Bus Selector/2 -> Heading/1  "<phi;theta;psi>"
  Velocity Conversion/1 -> Airspeed (kts)/1
  vt/1 -> Velocity Conversion/1
  Dot Product/1 -> vt/1
  Bus Selector/1 -> Dot Product/1, Dot Product/2  "<Vb>"
  Demands/1 -> Bus Selector/1
  Pitch Angle/1 -> Mux/2
  Bus Selector/5 -> PsiDot/1(Euler), Roll Angle/1, Pitch Angle/1  "<phi;theta;psi>"
  Demux2/3 -> PsiDot/3(r)  "r"
  Sideslip/1 -> Mux1/2  "beta"
  GaugeGain/1 -> Mux1/1
  Demux2/1 -> Terminator/1  "p"
  Demux2/2 -> PsiDot/2(q)  "q"
  Bus Selector/6 -> Demux2/1  "<pqr>"
  Bus Selector/7 -> Sideslip/1  "<Alpha;Beta>"
  PsiDot/1(psi_dot) -> GaugeGain/1
  Mux1/1 -> Angle Conversion/1
  Angle Conversion/1 -> "Turn, SlipSkid (deg)"/1

== system aeroblk_HL20_UE/Guidance System/Guide to Glideslope/Low Pass ==
  In1 : Inport
  Integrator : Integrator  InitialConditionSource=external
  Omega : Gain  Gain=2  SaturateOnIntegerOverflow=on  OutDataTypeStr=Inherit: Same as input  ParamDataTypeStr=Inherit: Same as input
  Sum3 : Sum  Inputs=|+-  InputSameDT=on  SaturateOnIntegerOverflow=on  OutDataTypeStr=Inherit: Same as first input
  Out1 : Outport  VectorParamsAs1DForOutWhenUnconnected=off
  wires:
  Omega/1 -> Integrator/1
  Sum3/1 -> Omega/1
  Integrator/1 -> Sum3/2, Out1/1
  In1/1 -> Sum3/1, Integrator/2

== system aeroblk_HL20_UE/UE Visualization/Actuator Breakout/Extended ==
  note: Set bones 49 - 57 to rest position
  Action Port : ActionPort  ActionPortLabel=else
  Constant : Constant  Value=zeros(9, 3)  VectorParams1D=off
  Out1 : Outport
  wires:
  Constant/1 -> Out1/1

== system aeroblk_HL20_UE/UE Visualization/Actuator Breakout/Retracted ==
  note: Set rotation for bones 49 - 57: nose gear (49), left main (52), right main (55)
  Action Port : ActionPort  ActionPortLabel=if(u1 > u2)
  Constant : Constant  Value=zeros(2, 3)  VectorParams1D=off
  Constant1 : Constant  Value=zeros(2, 3)  VectorParams1D=off
  Constant2 : Constant  Value=zeros(2, 3)  VectorParams1D=off
  Left Main : Constant  Value=[-2 0 0]  VectorParams1D=off
  Matrix Concatenate : Concatenate  NumInputs=6  Mode=Multidimensional array
  Nose Gear : Constant  Value=[0 0 1.75]  VectorParams1D=off
  Right Main : Constant  Value=[2 0 0]  VectorParams1D=off
  Out1 : Outport
  wires:
  Matrix Concatenate/1 -> Out1/1
  Constant/1 -> Matrix Concatenate/2
  Constant1/1 -> Matrix Concatenate/4
  Constant2/1 -> Matrix Concatenate/6
  Right Main/1 -> Matrix Concatenate/5
  Left Main/1 -> Matrix Concatenate/3
  Nose Gear/1 -> Matrix Concatenate/1

== system aeroblk_HL20_UE/UE Visualization/Extract Flight Instruments/PsiDot ==
  Euler : Inport
  q : Inport  Port=2
  r : Inport  Port=3
  Add : Sum
  Cos : Trigonometry  Operator=cos
  Demux : Demux  Outputs=3
  Product : Product  Inputs=**/
  Product1 : Product  Inputs=**/
  SinCos : Trigonometry  Operator=sincos
  Terminator : Terminator
  psi_dot : Outport
  wires:
  Euler/1 -> Demux/1
  Demux/3 -> Terminator/1
  SinCos/2 -> Product/1
  SinCos/1 -> Product1/1
  Product/1 -> Add/2
  Product1/1 -> Add/1
  r/1 -> Product/2
  q/1 -> Product1/2
  Cos/1 -> Product1/3, Product/3
  Add/1 -> psi_dot/1
  Demux/2 -> Cos/1  "theta"
  Demux/1 -> SinCos/1  "phi"
